simulink model "singlePendulum"  (R2022a)
settings: Solver=ode45  StartTime=0.0  StopTime=10  MaxStep=0.0001  RelTol=1e-4
undefined symbols (not defined in the file): a_x, a_y, omega_x, omega_y
settings Model: Creator=semen  LastModifiedBy=semen

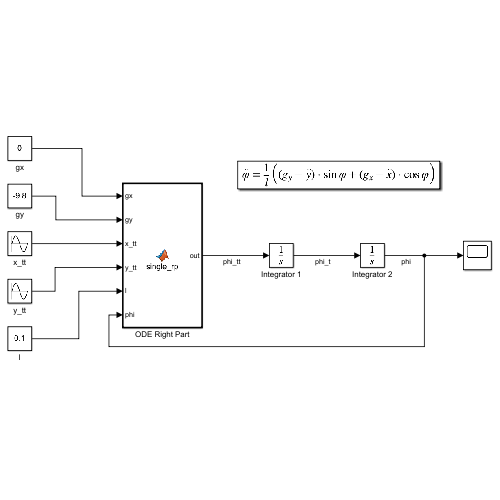
[thumbnail: Simulink's stored preview of the top-level diagram]
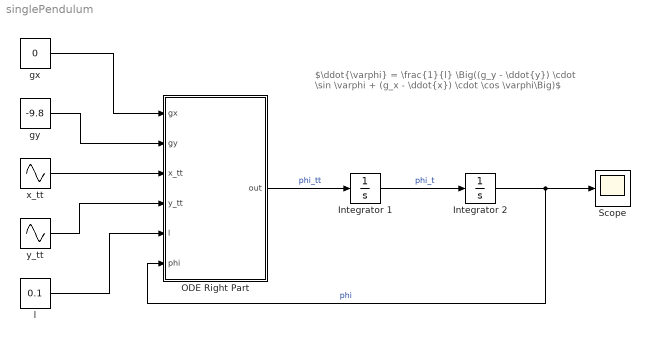
== system singlePendulum ==
  note: $\ddot{\varphi} = \frac{1}{l} \Big((g_y - \ddot{y}) \cdot \sin \varphi + (g_x - \ddot{x}) \cdot \cos \varphi\Big)$
  Integrator 1 : Integrator
  Integrator 2 : Integrator  InitialCondition=0.9 * pi
  ODE Right Part : MATLAB Function  TreatAsAtomicUnit=on
  Scope : Scope
  gx : Constant  Value=0
  gy : Constant  Value=-9.8
  l : Constant  Value=0.1
  x_tt : Sin  Amplitude=-a_x * omega_x ^ 2  Frequency=omega_x  SampleTime=0
  y_tt : Sin  Amplitude=-a_y * omega_y ^ 2  Frequency=omega_y  SampleTime=0
  wires:
  Integrator 1/1 -> Integrator 2/1  "phi_t"
  Integrator 2/1 -> Scope/1, ODE Right Part/6(phi)  "phi"
  ODE Right Part/1(out) -> Integrator 1/1  "phi_tt"
  gy/1 -> ODE Right Part/2(gy)
  gx/1 -> ODE Right Part/1(gx)
  l/1 -> ODE Right Part/5(l)
  x_tt/1 -> ODE Right Part/3(x_tt)
  y_tt/1 -> ODE Right Part/4(y_tt)

== matlab function singlePendulum/ODE Right Part ==
  data: gx input; out output; gy input; x_tt input; y_tt input; l input; phi input
function out = single_rp(gx, gy, x_tt, y_tt, l, phi)
    out = ((gx - x_tt) * cos(phi) + (gy - y_tt) * sin(phi)) / l;
end
